simulink model "FOC_PMSM_JugandonoslaConDong_cris_v13"  (R2019b)
settings: Solver=VariableStepAuto  StartTime=0  StopTime=1.5  FixedStep=1/fs/4  MaxStep=1/fs/2  RelTol=1e-7  EnableMultiTasking=on
InitFcn:
  | Motor_parameters_Lsrpm7fw
undefined symbols (not defined in the file): c2, DiscIntNeverNeededParam, fs, Iphmax, J, Ki1, Ki2, Ki3, Ki_pll, Kp1, Kp2, Kp3, Kp_pll, Ld, Lndd_ini, Lndmpm, Lq, Npp, Omegae_ini, Rs, sigbuilder_block, Tl_const, Trat, Vm, Vph, wo
libraries: simulink x2
settings Model: Creator=klu  LastModifiedBy=Kristina
settings DataIOCC: LimitDataPoints=on  SaveFormat=Array  SignalLoggingSaveFormat=ModelDataLogs  ReturnWorkspaceOutputs=off
settings OptimizationCC: BooleanDataType=off  ExpressionDepthLimit=2147483647  InitFltsAndDblsToZero=on  LifeSpan=inf
settings DebuggingCC: AlgebraicLoopMsg=none  SaveWithParameterizedLinksMsg=none  UnderspecifiedInitializationDetection=Classic  MergeDetectMultiDrivingBlocksExec=none  SignalResolutionControl=TryResolveAllWithWarning  MultiTaskDSMMsg=warning  MultiTaskCondExecSysMsg=none  FcnCallInpInsideContextMsg=warning  StateNameClashWarn=warning  SFUnexpectedBacktrackingDiag=warning  SFNoUnconditionalDefaultTransitionDiag=warning  SFExecutionAtInitializationDiag=none  ArithmeticOperatorsInVariantConditions=warning
settings HardwareCC: ProdBitPerPointer=32  ProdBitPerSizeT=32  ProdBitPerPtrDiffT=32  ProdLargestAtomicFloat=None  ProdIntDivRoundTo=Undefined  ProdEndianess=Unspecified  ProdWordSize=32  ProdHWDeviceType=32-bit Generic
settings ModelReferenceCC: PropagateSignalLabelsOutOfModel=off
settings SFSimCC: SimUseLocalCustomCode=off  CustomCodeUndefinedFunction=UseInterfaceOnly
settings RTWCC: RTWUseLocalCustomCode=off
settings CodeAppCC: StateflowObjectComments=on
settings GRTTargetCC: TargetFcnLib=ansi_tfl_tmw.mat  TargetLangStandard=C89/C90 (ANSI)  GeneratePreprocessorConditionals=Disable all  CombineOutputUpdateFcns=off  GRTInterface=on
settings ConfigComp: CovMetricSettings=dw  CovHtmlReporting=on  CovSaveCumulativeToWorkspaceVar=on  CovSaveSingleToWorkspaceVar=on  CovExternalEMLEnable=off  CovSFcnEnable=off

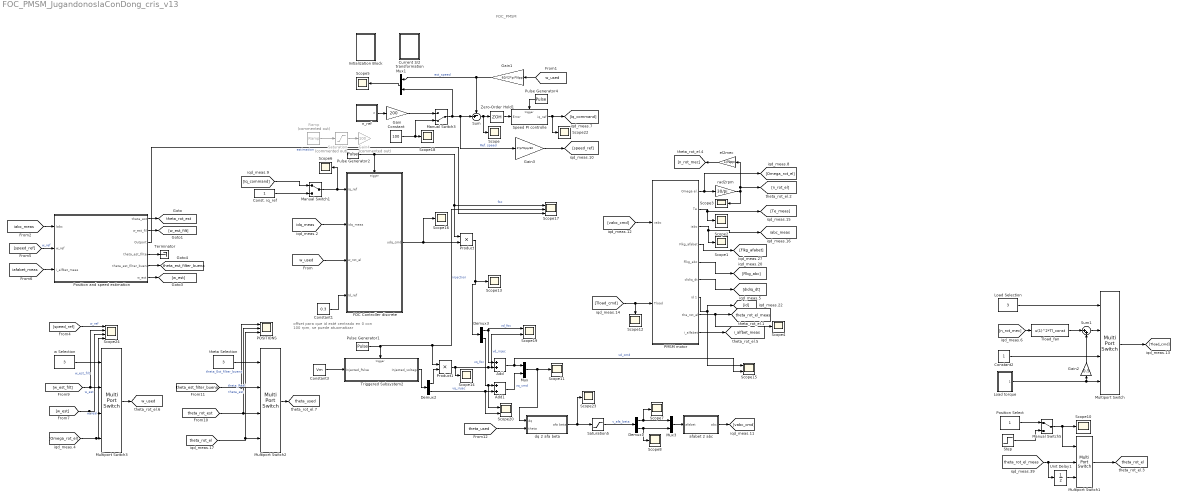
== system FOC_PMSM_JugandonoslaConDong_cris_v13 ==
  note: offset para que id esté centrado
      | en 0 con 100 rpm, se puede atuomatizar
  note: FOC_PMSM
  Add : Sum
  Add1 : Sum
  Const. iq_ref : Constant
  Constant : Constant  Value=100
  Constant1 : Constant  Value=0.3
  Constant2 : Constant
  Constant3 : Constant  Value=Vm
  Current 3/2 transformation : Subsystem
      mask Display:
      | plot([0.1000    0.1357    0.1714    0.2071    0.2429    0.2786    0.3143    0.3500    0.3857    0.4214 0.4571    0.4929    0.5286    0.5643    0.6000]-0.05,0.4+0.6*[0.5000    0.5868    0.6564    0.6950    0.6950    0.6564    0.5868    0.5000    0.4132    0.3436 0.3050    0.3050    0.3436    0.4132    0.5000])
      | 
      | plot([0.1,0.9],[0.1,0.9])
      | 
      | plot([0.5,0.9],0.3*[1 1])
  Demux1 : Demux  Outputs=2
  Demux2 : Demux  Outputs=2
  Demux3 : Demux  Outputs=2
  FOC Controller discrete : Subsystem
  Gain : Gain  Gain=200
  Gain1 : Gain  Gain=60/(2*pi*Npp)
  Gain2 : Gain  Gain=0.5
  Gain3 : Gain  Gain=2*pi*Npp/60
  Gain4 : Gain  Commented=on  Gain=100
  Initialization Block : Subsystem  mask{init_in=Motor_parameters_Lsrpm7fw}
      mask prompts: init_in "Enter Initialization Script:"
      mask init:
      | aaa =3;
      mask Callback init_in:
      | init_script=get_param(gcb,'MaskValueString');
      | %eval(init_script);
      | %set_param(gcs,'PreLoadFcn',init_script)
      | set_param(gcs,'InitFcn',init_script)
      | 
      | % Change the parameters here;
      | Ld               = Ld;
      | Lq               = Ld;
  Load Selection : Constant  Value=3
  Load torque : Subsystem
  Manual Switch1 : ManualSwitch
  Manual Switch3 : ManualSwitch  CurrentSetting=0
  Manual Switch5 : ManualSwitch
  Multiport Switch : MultiPortSwitch
  Multiport Switch1 : MultiPortSwitch  Inputs=2
  Multiport Switch2 : MultiPortSwitch
  Multiport Switch3 : MultiPortSwitch
  Mux : Mux  Inputs=2
  Mux1 : Mux  Inputs=2
  Mux3 : Mux  Inputs=2
  PMSM motor : Subsystem
  POSITIONS : Scope  NumInputPorts=3
  Position Select : Constant
  Position and speed estimation : Subsystem  TreatAsAtomicUnit=on
  Product : Product
  Product1 : Product
  Pulse Generator1 : DiscretePulseGenerator  PulseType=Time based  Period=2/fs  PulseWidth=50
  Pulse Generator2 : DiscretePulseGenerator  PulseType=Time based  Period=2/fs  PulseWidth=50  PhaseDelay=1/fs
  Pulse Generator4 : DiscretePulseGenerator  PulseType=Time based  Period=2/fs  PulseWidth=50  PhaseDelay=1/fs
  Ramp : simulink/Sources/Ramp  Commented=on  slope=0.5  start=0  InitialOutput=0.2
  Saturation : Saturate  Commented=on  UpperLimit=1
  Saturation5 : Saturate  UpperLimit=Vph  LowerLimit=-Vph
  Scope{,1..8,10..14,16,18,22..23} (18 alike) : Scope
  Scope15 : Scope  NumInputPorts=2
  Scope17 : Scope  NumInputPorts=3
  Scope19 : Scope  NumInputPorts=2
  Scope20 : Scope  NumInputPorts=2
  Scope24 : Scope  NumInputPorts=4
  Speed PI controlle : Subsystem
  Step : Step  Time=0  Before=1  After=2  SampleTime=0
  Sum : Sum  Inputs=-+|
  Sum1 : Sum  Inputs=|++
  Terminator : Terminator
  Tload_fan : Fcn  Expr=u(1)^2*Tl_const
  Triggered Subsystem2 : Subsystem  TreatAsAtomicUnit=on
  Unit Delay1 : UnitDelay  SampleTime=(1/fs)*4  HasFrameUpgradeWarning=on
  Zero-Order Hold1 : ZeroOrderHold  SampleTime=1/5e3
  afabet 2 abc : Subsystem
  dq 2 afa beta : Subsystem
  el2mec : Gain  Gain=1/Npp
  n_ref : Subsystem  Tag=STV Subsys  LoadFcn=sigbuilder_block('load');  StartFcn=sigbuilder_block('start');  StopFcn=sigbuilder_block('stop');  ClipboardFcn=sigbuilder_block('clipboard');  mask(Sigbuilder block){tuvar=[0:10]}
      mask help: Sigbuilder GUI
      mask init:
      | if ~strcmp(get_param(bdroot(gcbh),'SimulationStatus'),'stopped') tuvar = sigbuilder_block('maskInit'); end
      settings: CopyFcn=sigbuilder_block('copy');  DeleteFcn=sigbuilder_block('delete');  ModelCloseFcn=sigbuilder_block('modelClose');  PreSaveFcn=sigbuilder_block('preSave');  PauseFcn=sigbuilder_block('pause')  ContinueFcn=sigbuilder_block('continue')  NameChangeFcn=sigbuilder_block('namechange');  OpenFcn=sigbuilder_block('open',[72.75 116.25 550.5 363.75 ]);  CloseFcn=sigbuilder_block('close');
      mask Display: plot(0, 0, 100, 100,[2, 2, 32, 32, 2], [68, 8, 8, 68, 68],[32, 2], [38, 38], [32, 19, 2],[53, 60, 44], [32, 17, 17, 2],[16, 16, 31, 31]);txt = getActiveGroup(gcbh);text(2, 100, txt,'verticalAlignment', 'top');
  rad2rpm : Gain  Gain=30/pi
  theta Selection : Constant  Value=3
  w Selection : Constant  Value=3
  tag scope: i_alfbet_meas=global, iabc_meas=global, theta_est_filter_buena=global, theta_rot_el=global, theta_rot_el_meas=global, theta_rot_est=global, theta_used=global, w_used=global
  wires:
  Mux1/1 -> Scope5/1
  Sum/1 -> Scope/1, Zero-Order Hold1/1
  Manual Switch1/1 -> Scope6/1, FOC Controller discrete/1(iq_ref)
  Const. iq_ref/1 -> Manual Switch1/2
  Zero-Order Hold1/1 -> Speed PI controlle/1(Error)
  Constant/1 -> Manual Switch3/2, Scope18/1
  Manual Switch3/1 -> Mux1/2, Gain3/1, Sum/2  "Ref. speed"
  [idq_meas] -> FOC Controller discrete/2(idq_meas)
  Constant2/1 -> Multiport Switch/3
  Load torque/1(T_load) -> Multiport Switch/4, Gain2/1
  Multiport Switch/1 -> [Tload_cmd]
  [n_rot_mec] -> Tload_fan/1
  Load Selection/1 -> Multiport Switch/1
  [theta_rot_el_meas] -> Unit Delay1/1, Multiport Switch1/2
  Multiport Switch1/1 -> [theta_rot_el]
  Position Select/1 -> Manual Switch5/1
  Step/1 -> Manual Switch5/2
  Manual Switch5/1 -> Multiport Switch1/1, Scope10/1
  n_ref/1(n) -> Gain/1
  Gain/1 -> Manual Switch3/1
  Sum1/1 -> Multiport Switch/2
  Tload_fan/1 -> Sum1/1
  Pulse Generator4/1 -> Speed PI controlle/Trigger
  Constant1/1 -> FOC Controller discrete/4(Id_ref)
  Gain2/1 -> Sum1/2
  Unit Delay1/1 -> Multiport Switch1/3
  [vabc_cmd] -> PMSM motor/1(vabc)
  rad2rpm/1 -> el2mec/1, [n_rot_el], Scope3/1
  [Tload_cmd] -> PMSM motor/2(Tload), Scope12/1
  Demux1/2 -> Mux3/2, Scope8/1
  Demux1/1 -> Scope7/1, Mux3/1
  Saturation5/1 -> Demux1/1  "v_afa_beta"
  afabet 2 abc/1(abc) -> [vabc_cmd]
  Mux3/1 -> afabet 2 abc/1(afabet)
  el2mec/1 -> [n_rot_mec]
  Speed PI controlle/1(iq_ref) -> [Iq_command], Scope22/1
  [Iq_command] -> Manual Switch1/1
  Position and speed estimation/2(w_est_fil) -> [w_est_filt]
  Position and speed estimation/1(theta_est) -> [theta_rot_est]
  [iabc_meas] -> Position and speed estimation/1(Iabc)
  Gain1/1 -> Mux1/1, Sum/1  "est_speed"
  Gain3/1 -> [speed_ref]
  dq 2 afa beta/1(afa beta) -> Scope23/1, Saturation5/1
  [theta_used] -> dq 2 afa beta/2(theta)
  Constant3/1 -> Triggered Subsystem2/1(Injected_Pulse)
  FOC Controller discrete/1(udq_cmd) -> Product/2, Scope16/1
  Pulse Generator2/1 -> Product/1, Scope17/1, FOC Controller discrete/Trigger  "foc"
  Product/1 -> Scope13/1, Demux3/1
  Pulse Generator1/1 -> Scope17/2, Product1/1, Triggered Subsystem2/Trigger  "injection"
  Product1/1 -> Scope19/2, Add/2, Scope14/1  "vd_injec"
  Position and speed estimation/3(Outport) -> Scope17/3  "estimation"
  Triggered Subsystem2/1("Injected_voltage ") -> Demux2/1
  Demux2/1 -> Product1/2
  Demux3/1 -> Add/1, Scope19/1  "vd_foc"
  Demux2/2 -> Scope20/2, Add1/2  "vq_injec"
  Demux3/2 -> Scope20/1, Add1/1  "vq_foc"
  Add1/1 -> Mux/2  "vq_cmd"
  Mux/1 -> dq 2 afa beta/1(dq), Scope11/1
  Add/1 -> Scope15/2, Mux/1  "vd_cmd"
  Ramp/1 -> Saturation/1
  Saturation/1 -> Gain4/1
  PMSM motor/1(Omega el.) -> [Omega_rot_el], rad2rpm/1
  PMSM motor/2(Te) -> [Te_meas], Scope2/1
  PMSM motor/3(iabc) -> Scope1/1, [iabc_meas]
  PMSM motor/8(the_rot_el) -> Scope4/1, [theta_rot_el_meas]
  PMSM motor/7(id 1) -> [id], Scope15/1
  PMSM motor/6(didiq_dt) -> [didiq_dt]
  PMSM motor/5(Flkg_abc) -> [Flkg_abc]
  PMSM motor/4(Flkg_afabet) -> [Flkg_afabet]
  Position and speed estimation/4(theta_est_filter) -> Terminator/1
  Position and speed estimation/5(theta_est_filter_buena) -> [theta_est_filter_buena]
  PMSM motor/9(i_alfabet) -> [i_alfbet_meas]
  [iafabet_meas] -> Position and speed estimation/3(i_alfbet_meas)
  Position and speed estimation/6(w_est) -> [w_est]
  [w_used] -> Gain1/1
  [w_est_filt] -> Scope24/2, Multiport Switch3/2  "w_est_filt"
  [Omega_rot_el] -> Scope24/4, Multiport Switch3/4  "w_real"
  Multiport Switch3/1 -> [w_used]
  theta Selection/1 -> Multiport Switch2/1
  [theta_est_filter_buena] -> POSITIONS/1, Multiport Switch2/2  "theta_Est_filter_buena"
  [theta_rot_est] -> POSITIONS/2, Multiport Switch2/3  "theta_est"
  [theta_rot_el] -> POSITIONS/3, Multiport Switch2/4  "theta_Real"
  Multiport Switch2/1 -> [theta_used]
  w Selection/1 -> Multiport Switch3/1
  [w_est] -> Scope24/3, Multiport Switch3/3  "w_est"
  [speed_ref] -> Scope24/1  "w_ref"
  [speed_ref] -> Position and speed estimation/2(w_ref)  "w_ref"
  [w_used] -> FOC Controller discrete/3(w_rot_el)

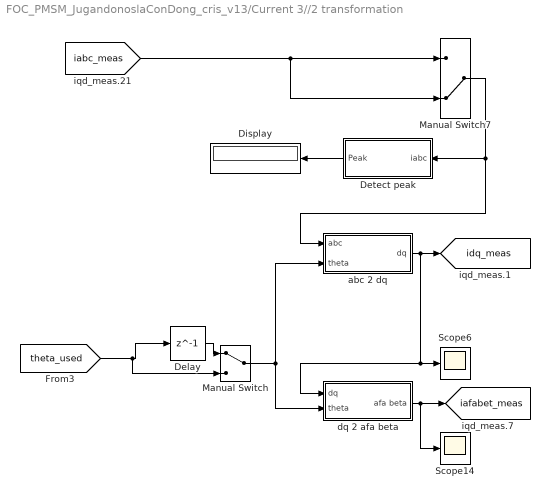
== system FOC_PMSM_JugandonoslaConDong_cris_v13/Current 3//2 transformation ==
  Delay : Delay  DelayLength=1
  Detect peak : Subsystem
  Display : Display
  Manual Switch : ManualSwitch
  Manual Switch7 : ManualSwitch  CurrentSetting=0
  Scope14 : Scope
  Scope6 : Scope
  abc 2 dq : Subsystem
  dq 2 afa beta : Subsystem
  tag scope: iafabet_meas=global, idq_meas=global
  wires:
  abc 2 dq/1(dq) -> [idq_meas], Scope6/1, dq 2 afa beta/1(dq)
  dq 2 afa beta/1(afa beta) -> [iafabet_meas], Scope14/1
  Manual Switch7/1 -> abc 2 dq/1(abc), Detect peak/1(iabc)
  Detect peak/1(Peak) -> Display/1
  [iabc_meas] -> Manual Switch7/1, Manual Switch7/2
  Manual Switch/1 -> abc 2 dq/2(theta), dq 2 afa beta/2(theta)
  Delay/1 -> Manual Switch/1
  [theta_used] -> Manual Switch/2, Delay/1

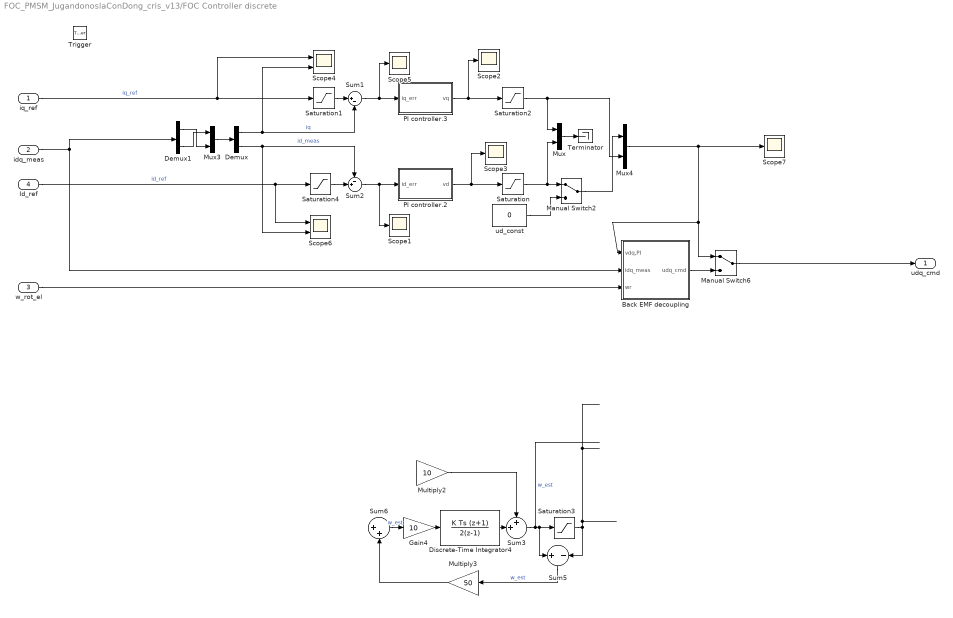
== system FOC_PMSM_JugandonoslaConDong_cris_v13/FOC Controller discrete ==
  iq_ref : Inport
  idq_meas : Inport  Port=2
  w_rot_el : Inport  Port=3
  Id_ref : Inport  Port=4
  Trigger : TriggerPort  VariantControl=(inherit)
  Back EMF decoupling : Subsystem
  Demux : Demux  Outputs=2
  Demux1 : Demux  Outputs=2
  Discrete-Time Integrator4 : DiscreteIntegrator  IntegratorMethod=Integration: Trapezoidal  gainval=1  SampleTime=-1  ICPrevOutput=DiscIntNeverNeededParam  ICPrevScaledInput=DiscIntNeverNeededParam
  Gain4 : Gain  Gain=10
  Manual Switch2 : ManualSwitch
  Manual Switch6 : ManualSwitch
  Multiply2 : Gain  Gain=10
  Multiply3 : Gain  Gain=50
  Mux : Mux  Inputs=2
  Mux3 : Mux  Inputs=2
  Mux4 : Mux  Inputs=2
  PI controller.2 : Subsystem
  PI controller.3 : Subsystem
  Saturation : Saturate  UpperLimit=Vph  LowerLimit=-Vph
  Saturation1 : Saturate  UpperLimit=Iphmax  LowerLimit=-Iphmax
  Saturation2 : Saturate  UpperLimit=Vph  LowerLimit=-Vph
  Saturation3 : Saturate  UpperLimit=110*Npp*2*pi/60
  Saturation4 : Saturate  UpperLimit=Iphmax  LowerLimit=-Iphmax
  Scope{1..3,5,7} (5 alike) : Scope
  Scope4 : Scope  NumInputPorts=2
  Scope6 : Scope  NumInputPorts=2
  Sum1 : Sum  Inputs=|+-
  Sum2 : Sum  Inputs=-+|
  Sum3 : Sum  Inputs=++|
  Sum5 : Sum  Inputs=+|-
  Sum6 : Sum  Inputs=|++
  Terminator : Terminator
  ud_const : Constant  Value=0
  udq_cmd : Outport  VectorParamsAs1DForOutWhenUnconnected=off
  wires:
  Saturation4/1 -> Sum2/2
  Saturation/1 -> Mux/2, Manual Switch2/1
  Mux/1 -> Terminator/1
  PI controller.3/1(vq) -> Scope2/1, Saturation2/1
  Demux/1 -> Scope4/2, Sum1/2  "iq"
  PI controller.2/1(vd) -> Saturation/1, Scope3/1
  Demux/2 -> Scope6/2, Sum2/1  "id_meas"
  Sum1/1 -> Scope5/1, PI controller.3/1(iq_err)
  iq_ref/1 -> Scope4/1, Saturation1/1  "iq_ref"
  Sum2/1 -> Scope1/1, PI controller.2/1(id_err)
  Id_ref/1 -> Scope6/1, Saturation4/1  "id_ref"
  Saturation1/1 -> Sum1/1
  Saturation2/1 -> Mux/1, Mux4/2
  Manual Switch2/1 -> Mux4/1
  ud_const/1 -> Manual Switch2/2
  Demux1/2 -> Mux3/1
  Demux1/1 -> Mux3/2
  w_rot_el/1 -> Back EMF decoupling/3(wr)
  Back EMF decoupling/1(udq_cmd) -> Manual Switch6/2
  Mux4/1 -> Scope7/1, Manual Switch6/1, Back EMF decoupling/1(vdq,PI)
  Mux3/1 -> Demux/1
  idq_meas/1 -> Demux1/1, Back EMF decoupling/2(idq_meas)
  Manual Switch6/1 -> udq_cmd/1
  Sum3/1 -> Sum5/1, Saturation3/1  "w_est"
  Saturation3/1 -> Sum5/2
  Sum6/1 -> Gain4/1  "w_est"
  Multiply3/1 -> Sum6/2
  ? -> Multiply2/1, Sum6/1  "theta_er"
  Gain4/1 -> Discrete-Time Integrator4/1
  Multiply2/1 -> Sum3/1
  Discrete-Time Integrator4/1 -> Sum3/2
  Sum5/1 -> Multiply3/1  "w_est"

== system FOC_PMSM_JugandonoslaConDong_cris_v13/Initialization Block ==

== system FOC_PMSM_JugandonoslaConDong_cris_v13/Load torque ==
  Add : Sum  Inputs=+++
  Scope2 : Scope
  Step Load torque 1 : Step  Time=0.7  After=Trat  SampleTime=0
  Step Load torque2 : Step  Time=2.5  After=-Trat  SampleTime=0
  Tload : Constant  Value=0
  T_load : Outport  VectorParamsAs1DForOutWhenUnconnected=off
  wires:
  Tload/1 -> Add/1
  Step Load torque 1/1 -> Add/2
  Step Load torque2/1 -> Add/3
  Add/1 -> T_load/1, Scope2/1

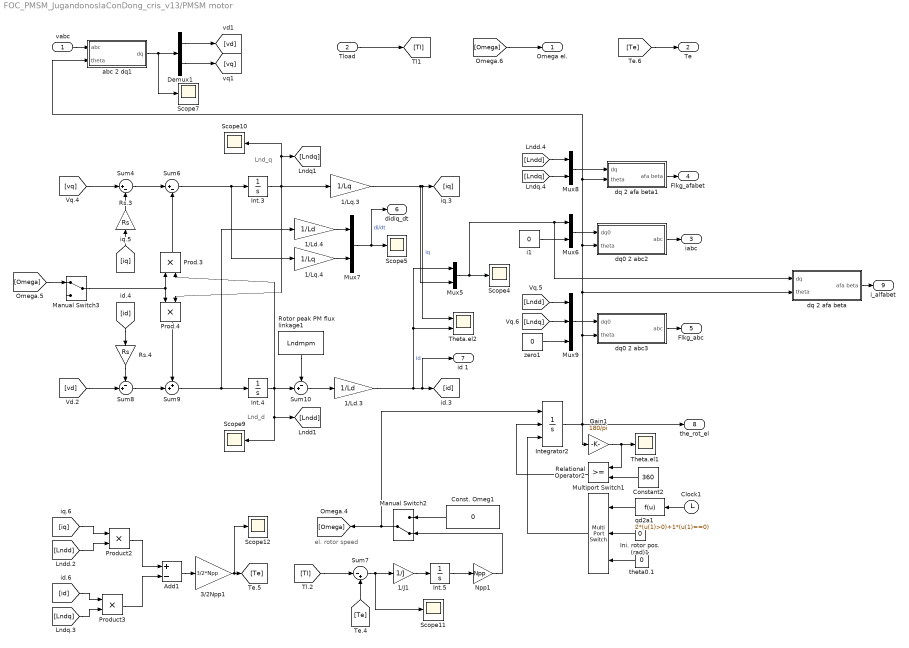
== system FOC_PMSM_JugandonoslaConDong_cris_v13/PMSM motor ==
  note: Lnd_d
  note: el. rotor speed
  note: Lnd_q
  vabc : Inport
  Tload : Inport  Port=2
  1/J1 : Gain  Gain=1/J
  1/Ld.3 : Gain  Gain=1/Ld
  1/Ld.4 : Gain  Gain=1/Ld
  1/Lq.3 : Gain  Gain=1/Lq
  1/Lq.4 : Gain  Gain=1/Lq
  3/2Npp1 : Gain  Gain=3/2*Npp
  Add1 : Sum  Inputs=+-
  Clock1 : Clock
  Const. Omeg1 : Constant  Value=0
  Constant2 : Constant  Value=360
  Demux1 : Demux  Outputs=2
  Gain1 : Gain  Gain=180/pi
  Ini. rotor pos. (rad)1 : Constant  Value=0
  Int.3 : Integrator
  Int.4 : Integrator  InitialCondition=Lndd_ini
  Int.5 : Integrator  InitialCondition=Omegae_ini/Npp
  Integrator2 : Integrator  ExternalReset=rising  InitialConditionSource=external  InitialCondition=pi/3
  Manual Switch2 : ManualSwitch  CurrentSetting=0
  Manual Switch3 : ManualSwitch
  Multiport Switch1 : MultiPortSwitch  Inputs=2
  Mux{5..8} (4 alike) : Mux  Inputs=2
  Mux9 : Mux  Inputs=3
  Npp1 : Gain  Gain=Npp
  Prod.3 : Product  RndMeth=Zero
  Prod.4 : Product  RndMeth=Zero
  Product2 : Product  RndMeth=Zero
  Product3 : Product  RndMeth=Zero
  Relational Operator2 : RelationalOperator  OutDataTypeStr=boolean  RndMeth=Nearest
  Rotor peak PM flux linkage1 : Constant  Value=Lndmpm
  Rs.3 : Gain  Gain=Rs
  Rs.4 : Gain  Gain=Rs
  Scope{4..5,7,9..12} (7 alike) : Scope
  Sum10 : Sum  Inputs=-+|
  Sum4 : Sum  Inputs=|+-
  Sum6 : Sum  Inputs=|+-
  Sum7 : Sum  Inputs=|-+
  Sum8 : Sum  Inputs=-+|
  Sum9 : Sum  Inputs=++|
  Theta.el1 : Scope
  Theta.el2 : Scope  NumInputPorts=2
  abc 2 dq1 : Subsystem
  dq 2 afa beta : Subsystem
  dq 2 afa beta1 : Subsystem
  dq0 2 abc2 : Subsystem
  dq0 2 abc3 : Subsystem
  i1 : Constant  Value=0
  qd2a1 : Fcn  Expr=2*(u(1)>0)+1*(u(1)==0)
  theta0.1 : Constant  Value=0
  zero1 : Constant  Value=0
  Omega el. : Outport  VectorParamsAs1DForOutWhenUnconnected=off
  Te : Outport  Port=2  VectorParamsAs1DForOutWhenUnconnected=off
  iabc : Outport  Port=3  VectorParamsAs1DForOutWhenUnconnected=off
  Flkg_afabet : Outport  Port=4  VectorParamsAs1DForOutWhenUnconnected=off
  Flkg_abc : Outport  Port=5  VectorParamsAs1DForOutWhenUnconnected=off
  didiq_dt : Outport  Port=6  VectorParamsAs1DForOutWhenUnconnected=off
  id 1 : Outport  Port=7  VectorParamsAs1DForOutWhenUnconnected=off
  the_rot_el : Outport  Port=8  VectorParamsAs1DForOutWhenUnconnected=off
  i_alfabet : Outport  Port=9  VectorParamsAs1DForOutWhenUnconnected=off
  wires:
  Sum4/1 -> Sum6/1
  [vd] -> Sum8/2
  Mux5/1 -> Scope4/1, dq 2 afa beta/1(dq), Mux6/1
  Mux7/1 -> didiq_dt/1, Scope5/1  "di/dt"
  Int.3/1 -> 1/Lq.3/1, Prod.4/2, Scope10/1, [Lndq]
  abc 2 dq1/1(dq) -> Demux1/1, Scope7/1
  Tload/1 -> [Tl]
  Rs.3/1 -> Sum4/2
  1/Ld.4/1 -> Mux7/1
  Integrator2/1 -> the_rot_el/1, dq 2 afa beta/2(theta), dq0 2 abc2/2(theta), dq 2 afa beta1/2(theta), abc 2 dq1/2(theta), dq0 2 abc3/2(theta), Gain1/1
  Prod.4/1 -> Sum9/1
  [Lndq] -> Product3/2
  1/J1/1 -> Int.5/1
  [Lndd] -> Mux8/1
  [Te] -> Te/1
  [iq] -> Rs.3/1
  Sum10/1 -> 1/Ld.3/1
  Rotor peak PM flux linkage1/1 -> Sum10/1
  Int.4/1 -> [Lndd], Scope9/1, Sum10/2, Prod.3/2
  Int.5/1 -> Npp1/1
  Sum8/1 -> Sum9/2
  Add1/1 -> 3/2Npp1/1
  3/2Npp1/1 -> Scope12/1, [Te]
  Product3/1 -> Add1/2
  Demux1/2 -> [vq]
  Prod.3/1 -> Sum6/2
  1/Lq.3/1 -> Theta.el2/1, [iq], Mux5/2  "iq"
  1/Ld.3/1 -> Theta.el2/2, Mux5/1, id 1/1, [id]  "id"
  [Omega] -> Omega el./1
  [Omega] -> Manual Switch3/1
  1/Lq.4/1 -> Mux7/2
  [vq] -> Sum4/1
  Npp1/1 -> Manual Switch2/2
  Gain1/1 -> Theta.el1/1, Relational Operator2/1
  dq0 2 abc2/1(abc) -> iabc/1
  [Te] -> Sum7/2
  Ini. rotor pos. (rad)1/1 -> Multiport Switch1/2
  Sum6/1 -> Int.3/1, 1/Lq.4/1
  Manual Switch3/1 -> Prod.4/1, Prod.3/1
  i1/1 -> Mux6/2
  dq0 2 abc3/1(abc) -> Flkg_abc/1
  Relational Operator2/1 -> Integrator2/2
  [Lndq] -> Mux9/2
  Multiport Switch1/1 -> Integrator2/3
  Constant2/1 -> Relational Operator2/2
  [Lndd] -> Product2/2
  [iq] -> Product2/1
  [id] -> Product3/1
  Product2/1 -> Add1/1
  Clock1/1 -> qd2a1/1
  [id] -> Rs.4/1
  vabc/1 -> abc 2 dq1/1(abc)
  Mux6/1 -> dq0 2 abc2/1(dq0)
  Demux1/1 -> [vd]
  Const. Omeg1/1 -> Manual Switch2/1
  Rs.4/1 -> Sum8/1
  [Lndd] -> Mux9/1
  theta0.1/1 -> Multiport Switch1/3
  Sum7/1 -> Scope11/1, 1/J1/1
  [Lndq] -> Mux8/2
  Mux9/1 -> dq0 2 abc3/1(dq0)
  Manual Switch2/1 -> Integrator2/1, [Omega]
  Mux8/1 -> dq 2 afa beta1/1(dq)
  dq 2 afa beta1/1(afa beta) -> Flkg_afabet/1
  qd2a1/1 -> Multiport Switch1/1
  zero1/1 -> Mux9/3
  [Tl] -> Sum7/1
  Sum9/1 -> Int.4/1, 1/Ld.4/1
  dq 2 afa beta/1(afa beta) -> i_alfabet/1

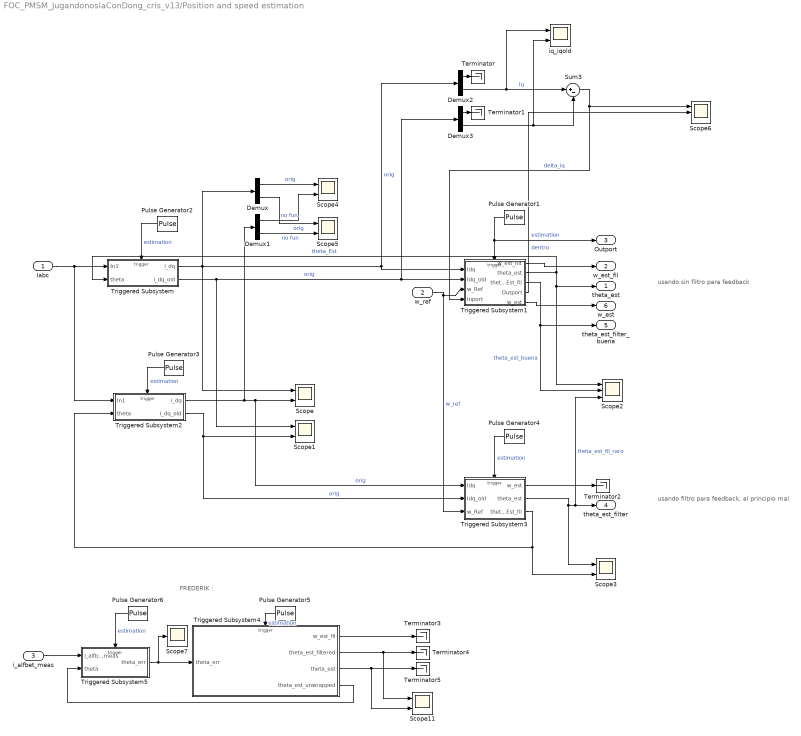
== system FOC_PMSM_JugandonoslaConDong_cris_v13/Position and speed estimation ==
  note: FREDERIK :
  note: usando filtro para feedback, al principio mal
  note: usando sin filtro para feedback
  Iabc : Inport
  w_ref : Inport  Port=2
  i_alfbet_meas : Inport  Port=3
  Demux{,1..3} (4 alike) : Demux  Outputs=2
  Pulse Generator1 : DiscretePulseGenerator  PulseType=Time based  Period=2/fs  PulseWidth=50
  Pulse Generator2 : DiscretePulseGenerator  PulseType=Time based  Period=1/fs  PulseWidth=50
  Pulse Generator3 : DiscretePulseGenerator  PulseType=Time based  Period=1/fs  PulseWidth=50
  Pulse Generator4 : DiscretePulseGenerator  PulseType=Time based  Period=2/fs  PulseWidth=50  PhaseDelay=1/fs
  Pulse Generator5 : DiscretePulseGenerator  PulseType=Time based  Period=2/fs  PulseWidth=50  PhaseDelay=1/fs
  Pulse Generator6 : DiscretePulseGenerator  PulseType=Time based  Period=1/fs  PulseWidth=50
  Scope{,1,3..5,11} (6 alike) : Scope  NumInputPorts=2
  Scope2 : Scope  NumInputPorts=3
  Scope6 : Scope  NumInputPorts=3
  Scope7 : Scope
  Sum3 : Sum  Inputs=|+-
  Terminator{,1..5} (6 alike) : Terminator
  Triggered Subsystem : Subsystem  TreatAsAtomicUnit=on
  Triggered Subsystem1 : Subsystem  TreatAsAtomicUnit=on
  Triggered Subsystem2 : Subsystem  TreatAsAtomicUnit=on
  Triggered Subsystem3 : Subsystem  TreatAsAtomicUnit=on
  Triggered Subsystem4 : Subsystem  TreatAsAtomicUnit=on
  Triggered Subsystem5 : Subsystem  TreatAsAtomicUnit=on
  iq_iqold : Scope  NumInputPorts=2
  theta_est : Outport
  w_est_fil : Outport  Port=2
  Outport : Outport  Port=3
  theta_est_filter : Outport  Port=4
  theta_est_filter_buena : Outport  Port=5
  w_est : Outport  Port=6
  wires:
  Pulse Generator1/1 -> Triggered Subsystem1/Trigger, Outport/1  "estimation"
  Triggered Subsystem1/1(w_est_filt) -> w_est_fil/1
  Triggered Subsystem/2(i_dq_old) -> Scope1/1, Demux3/1, Triggered Subsystem1/2(Idq_old)  "orig"
  Triggered Subsystem1/2(theta_est) -> Scope2/1, theta_est/1, Triggered Subsystem/2(theta)  "theta_Est"
  Triggered Subsystem/1(i_dq) -> Scope/1, Demux/1, Demux2/1, Triggered Subsystem1/1(Idq)  "orig"
  w_ref/1 -> Triggered Subsystem3/3(w_Ref), Triggered Subsystem1/3(w_Ref)  "w_ref"
  Pulse Generator2/1 -> Triggered Subsystem/Trigger  "estimation"
  Triggered Subsystem1/3(theta_Est_fil) -> theta_est_filter_buena/1, Scope2/2  "theta_est_buena"
  Pulse Generator3/1 -> Triggered Subsystem2/Trigger  "estimation"
  Demux/1 -> Scope4/1  "orig"
  Demux1/1 -> Scope4/2  "no fun"
  Demux/2 -> Scope5/1  "orig"
  Demux1/2 -> Scope5/2  "no fun"
  Pulse Generator4/1 -> Triggered Subsystem3/Trigger  "estimation"
  Triggered Subsystem3/3(theta_Est_fil) -> Triggered Subsystem2/2(theta), Scope3/2
  Triggered Subsystem2/2(i_dq_old) -> Triggered Subsystem3/2(Idq_old), Scope1/2  "orig"
  Triggered Subsystem2/1(i_dq) -> Triggered Subsystem3/1(Idq), Scope/2, Demux1/1  "orig"
  Triggered Subsystem3/2(theta_est) -> Scope3/1, Scope2/3, theta_est_filter/1  "theta_est_fil_raro"
  Triggered Subsystem3/1(w_est) -> Terminator2/1
  Demux2/1 -> Terminator/1
  Demux3/1 -> Terminator1/1
  Demux2/2 -> iq_iqold/1, Sum3/1  "Iq"
  Demux3/2 -> iq_iqold/2, Sum3/2
  Sum3/1 -> Triggered Subsystem1/4(Inport), Scope6/1  "delta_iq"
  Triggered Subsystem1/4(Outport) -> Scope6/2  "dentro"
  Iabc/1 -> Triggered Subsystem2/1(In1), Triggered Subsystem/1(In1)
  Triggered Subsystem4/3(theta_est) -> Terminator5/1, Scope11/2
  i_alfbet_meas/1 -> Triggered Subsystem5/1(i_alfbet_meas)
  Triggered Subsystem4/1(w_est_fil) -> Terminator3/1
  Triggered Subsystem4/2(theta_est_filtered) -> Terminator4/1, Scope11/1
  Pulse Generator5/1 -> Triggered Subsystem4/Trigger  "estimation"
  Pulse Generator6/1 -> Triggered Subsystem5/Trigger  "estimation"
  Triggered Subsystem5/1(theta_err) -> Scope7/1, Triggered Subsystem4/1(theta_err)
  Triggered Subsystem4/4(theta_est_unwrapped) -> Triggered Subsystem5/2(theta)
  Triggered Subsystem1/5(w_est) -> w_est/1

== system FOC_PMSM_JugandonoslaConDong_cris_v13/Speed PI controlle ==
  Error : Inport
  Trigger : TriggerPort  VariantControl=(inherit)
  Discrete-Time Integrator : DiscreteIntegrator  IntegratorMethod=Integration: Trapezoidal  SampleTime=-1  ICPrevOutput=DiscIntNeverNeededParam  ICPrevScaledInput=DiscIntNeverNeededParam
  Kp : Gain  Gain=Kp1
  Sum1 : Sum  Inputs=|++
  ki : Gain  Gain=Ki1
  iq_ref : Outport  VectorParamsAs1DForOutWhenUnconnected=off
  wires:
  Kp/1 -> Sum1/1
  ki/1 -> Discrete-Time Integrator/1
  Discrete-Time Integrator/1 -> Sum1/2
  Sum1/1 -> iq_ref/1
  Error/1 -> Kp/1, ki/1

== system FOC_PMSM_JugandonoslaConDong_cris_v13/Triggered Subsystem2 ==
  Injected_Pulse : Inport
  Trigger : TriggerPort  VariantControl=Variant
  Constant : Constant  Value=0
  Mux5 : Mux  Inputs=2
  Saturation3 : Saturate  UpperLimit=Vph  LowerLimit=-Vph
  "Injected_voltage " : Outport
  wires:
  Injected_Pulse/1 -> Mux5/1
  Constant/1 -> Mux5/2
  Mux5/1 -> Saturation3/1  "vdq_cmd_inj"
  Saturation3/1 -> "Injected_voltage "/1

== system FOC_PMSM_JugandonoslaConDong_cris_v13/afabet 2 abc ==
  afabet : Inport
  Constant : Constant  Value=0
  Mux1 : Mux  Inputs=2
  Mux2 : Mux  Inputs=3
  qd2a : Fcn  Expr=u(1)+u(3)
  qd2b : Fcn  Expr=u(1)*cos(2/3*pi)+u(2)*sin(2/3*pi)+u(3)
  qd2c : Fcn  Expr=u(1)*cos(2/3*pi)-u(2)*sin(2/3*pi)+u(3)
  abc : Outport  VectorParamsAs1DForOutWhenUnconnected=off
  wires:
  Constant/1 -> Mux1/2
  qd2c/1 -> Mux2/3
  afabet/1 -> Mux1/1
  Mux1/1 -> qd2c/1, qd2b/1, qd2a/1
  qd2a/1 -> Mux2/1
  qd2b/1 -> Mux2/2
  Mux2/1 -> abc/1

== system FOC_PMSM_JugandonoslaConDong_cris_v13/dq 2 afa beta ==
  dq : Inport
  theta : Inport  Port=2
  Mux1 : Mux  Inputs=2
  Mux2 : Mux  Inputs=2
  dq2afa : Fcn  Expr=u(1)*cos(u(3))-u(2)*sin(u(3))
  dq2beta : Fcn  Expr=u(1)*sin(u(3))+u(2)*cos(u(3))
  afa beta : Outport  VectorParamsAs1DForOutWhenUnconnected=off
  wires:
  Mux2/1 -> afa beta/1
  dq2beta/1 -> Mux2/2
  dq2afa/1 -> Mux2/1
  Mux1/1 -> dq2afa/1, dq2beta/1
  theta/1 -> Mux1/2
  dq/1 -> Mux1/1

== system FOC_PMSM_JugandonoslaConDong_cris_v13/n_ref ==
  Demux : Demux  Tag=STV Demux  Outputs=1
  FromWs : FromWorkspace  Tag=STV FromWs  VariableName=tuvar  SampleTime=0
      SigBuilderData=|
      | common.afterFinalStr = 'Extrapolate'
      | common.sampleTime = 0
      | dataSet.timeRange = [0 10]
      | dataSet.name = 'Group 1'
      | sbobj.Groups.Name = 'Group 1'
      | sbobj.Groups.Signals.Name = 'n'
      | sbobj.Groups.Signals.XData = [0 4 4 5 5 7 10]
      | sbobj.Groups.Signals.YData = [0.21 0.795 0.995 0.995 0.4 0.405 0.2]
  n : Outport  Tag=STV Outport  VectorParamsAs1DForOutWhenUnconnected=off
  wires:
  Demux/1 -> n/1
  FromWs/1 -> Demux/1

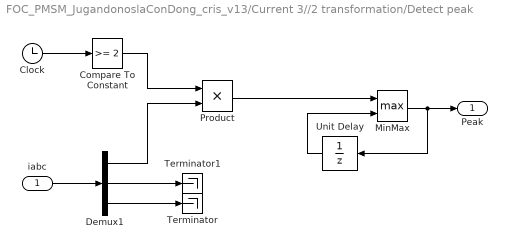
== system FOC_PMSM_JugandonoslaConDong_cris_v13/Current 3//2 transformation/Detect peak ==
  iabc : Inport
  Clock : Clock
  Compare To Constant : simulink/Logic and Bit Operations/Compare To Constant  relop=>=  const=2  OutDataTypeStr=uint8  ZeroCross=off
  Demux1 : Demux  Outputs=3
  MinMax : MinMax  Function=max  Inputs=2
  Product : Product  RndMeth=Zero
  Terminator : Terminator
  Terminator1 : Terminator
  Unit Delay : UnitDelay  SampleTime=1/5e3  HasFrameUpgradeWarning=on
  Peak : Outport  VectorParamsAs1DForOutWhenUnconnected=off
  wires:
  iabc/1 -> Demux1/1
  Demux1/3 -> Terminator/1
  Demux1/2 -> Terminator1/1
  Clock/1 -> Compare To Constant/1
  Compare To Constant/1 -> Product/1
  Demux1/1 -> Product/2
  MinMax/1 -> Peak/1, Unit Delay/1
  Product/1 -> MinMax/1
  Unit Delay/1 -> MinMax/2

== system FOC_PMSM_JugandonoslaConDong_cris_v13/Current 3//2 transformation/abc 2 dq ==
  abc : Inport
  theta : Inport  Port=2
  Mux1 : Mux  Inputs=2
  Mux2 : Mux  Inputs=2
  abc2d : Fcn  Expr=2/3*(u(1)*cos(u(4))+u(2)*cos(u(4)-2*pi/3)+u(3)*cos(u(4)-4*pi/3))
  abc2q : Fcn  Expr=-1*2/3*(u(1)*sin(u(4))+u(2)*sin(u(4)-2*pi/3)+u(3)*sin(u(4)-4*pi/3))
  dq : Outport  VectorParamsAs1DForOutWhenUnconnected=off
  wires:
  Mux2/1 -> dq/1
  abc2q/1 -> Mux2/2
  abc2d/1 -> Mux2/1
  Mux1/1 -> abc2q/1, abc2d/1
  theta/1 -> Mux1/2
  abc/1 -> Mux1/1

== system FOC_PMSM_JugandonoslaConDong_cris_v13/Current 3//2 transformation/dq 2 afa beta ==
  dq : Inport
  theta : Inport  Port=2
  Mux1 : Mux  Inputs=2
  Mux2 : Mux  Inputs=2
  dq2afa : Fcn  Expr=u(1)*cos(u(3))-u(2)*sin(u(3))
  dq2beta : Fcn  Expr=u(1)*sin(u(3))+u(2)*cos(u(3))
  afa beta : Outport  VectorParamsAs1DForOutWhenUnconnected=off
  wires:
  dq/1 -> Mux1/1
  theta/1 -> Mux1/2
  Mux1/1 -> dq2beta/1, dq2afa/1
  dq2afa/1 -> Mux2/1
  dq2beta/1 -> Mux2/2
  Mux2/1 -> afa beta/1

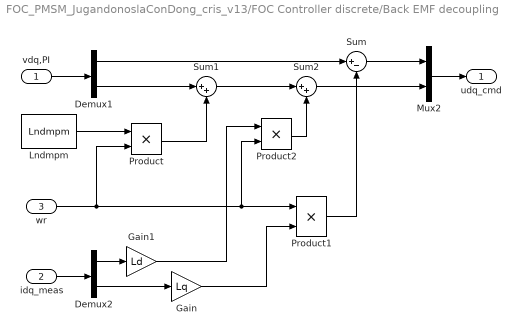
== system FOC_PMSM_JugandonoslaConDong_cris_v13/FOC Controller discrete/Back EMF decoupling ==
  vdq,PI : Inport
  idq_meas : Inport  Port=2
  wr : Inport  Port=3
  Demux1 : Demux  Outputs=2
  Demux2 : Demux  Outputs=2
  Gain : Gain  Gain=Lq
  Gain1 : Gain  Gain=Ld
  Lndmpm : Constant  Value=Lndmpm
  Mux2 : Mux  Inputs=2
  Product : Product  RndMeth=Zero
  Product1 : Product  RndMeth=Zero
  Product2 : Product  RndMeth=Zero
  Sum : Sum  Inputs=|+-
  Sum1 : Sum  Inputs=|++
  Sum2 : Sum  Inputs=|++
  udq_cmd : Outport  VectorParamsAs1DForOutWhenUnconnected=off
  wires:
  Mux2/1 -> udq_cmd/1
  vdq,PI/1 -> Demux1/1
  Demux1/1 -> Sum/1
  Sum/1 -> Mux2/1
  Demux1/2 -> Sum1/1
  idq_meas/1 -> Demux2/1
  wr/1 -> Product/2, Product1/1, Product2/2
  Product1/1 -> Sum/2
  Gain/1 -> Product1/2
  Demux2/2 -> Gain/1
  Lndmpm/1 -> Product/1
  Product/1 -> Sum1/2
  Sum1/1 -> Sum2/1
  Demux2/1 -> Gain1/1
  Gain1/1 -> Product2/1
  Product2/1 -> Sum2/2
  Sum2/1 -> Mux2/2

== system FOC_PMSM_JugandonoslaConDong_cris_v13/FOC Controller discrete/PI controller.2 ==
  id_err : Inport
  Discrete-Time Integrator : DiscreteIntegrator  IntegratorMethod=Integration: Trapezoidal  SampleTime=-1  ICPrevOutput=DiscIntNeverNeededParam  ICPrevScaledInput=DiscIntNeverNeededParam
  Kp : Gain  Gain=Kp2
  Sum1 : Sum  Inputs=|++
  ki : Gain  Gain=Ki2
  vd : Outport  VectorParamsAs1DForOutWhenUnconnected=off
  wires:
  Sum1/1 -> vd/1
  Discrete-Time Integrator/1 -> Sum1/2
  ki/1 -> Discrete-Time Integrator/1
  Kp/1 -> Sum1/1
  id_err/1 -> ki/1, Kp/1

== system FOC_PMSM_JugandonoslaConDong_cris_v13/FOC Controller discrete/PI controller.3 ==
  iq_err : Inport
  Discrete-Time Integrator : DiscreteIntegrator  IntegratorMethod=Integration: Trapezoidal  SampleTime=-1  ICPrevOutput=DiscIntNeverNeededParam  ICPrevScaledInput=DiscIntNeverNeededParam
  Kp : Gain  Gain=Kp3
  Sum1 : Sum  Inputs=|++
  ki : Gain  Gain=Ki3
  vq : Outport  VectorParamsAs1DForOutWhenUnconnected=off
  wires:
  Sum1/1 -> vq/1
  Discrete-Time Integrator/1 -> Sum1/2
  ki/1 -> Discrete-Time Integrator/1
  Kp/1 -> Sum1/1
  iq_err/1 -> ki/1, Kp/1

== system FOC_PMSM_JugandonoslaConDong_cris_v13/PMSM motor/abc 2 dq1 ==
  abc : Inport
  theta : Inport  Port=2
  Mux1 : Mux  Inputs=2
  Mux2 : Mux  Inputs=2
  abc2d : Fcn  Expr=-1*2/3*(u(1)*sin(u(4))+u(2)*sin(u(4)-2*pi/3)+u(3)*sin(u(4)-4*pi/3))
  abc2q : Fcn  Expr=2/3*(u(1)*cos(u(4))+u(2)*cos(u(4)-2*pi/3)+u(3)*cos(u(4)-4*pi/3))
  dq : Outport  VectorParamsAs1DForOutWhenUnconnected=off
  wires:
  Mux2/1 -> dq/1
  abc2d/1 -> Mux2/2
  abc2q/1 -> Mux2/1
  Mux1/1 -> abc2d/1, abc2q/1
  theta/1 -> Mux1/2
  abc/1 -> Mux1/1

== system FOC_PMSM_JugandonoslaConDong_cris_v13/PMSM motor/dq 2 afa beta ==
  dq : Inport
  theta : Inport  Port=2
  Mux1 : Mux  Inputs=2
  Mux2 : Mux  Inputs=2
  dq2afa : Fcn  Expr=u(1)*cos(u(3))-u(2)*sin(u(3))
  dq2beta : Fcn  Expr=u(1)*sin(u(3))+u(2)*cos(u(3))
  afa beta : Outport  VectorParamsAs1DForOutWhenUnconnected=off
  wires:
  Mux2/1 -> afa beta/1
  dq2beta/1 -> Mux2/2
  dq2afa/1 -> Mux2/1
  Mux1/1 -> dq2afa/1, dq2beta/1
  theta/1 -> Mux1/2
  dq/1 -> Mux1/1

== system FOC_PMSM_JugandonoslaConDong_cris_v13/PMSM motor/dq 2 afa beta1 ==
  dq : Inport
  theta : Inport  Port=2
  Mux1 : Mux  Inputs=2
  Mux2 : Mux  Inputs=2
  dq2afa : Fcn  Expr=u(1)*cos(u(3))-u(2)*sin(u(3))
  dq2beta : Fcn  Expr=u(1)*sin(u(3))+u(2)*cos(u(3))
  afa beta : Outport  VectorParamsAs1DForOutWhenUnconnected=off
  wires:
  dq/1 -> Mux1/1
  theta/1 -> Mux1/2
  Mux1/1 -> dq2beta/1, dq2afa/1
  dq2afa/1 -> Mux2/1
  dq2beta/1 -> Mux2/2
  Mux2/1 -> afa beta/1

== system FOC_PMSM_JugandonoslaConDong_cris_v13/PMSM motor/dq0 2 abc2 ==
  dq0 : Inport
  theta : Inport  Port=2
  Mux1 : Mux  Inputs=2
  Mux2 : Mux  Inputs=3
  qd2a : Fcn  Expr=u(1)*cos(u(4))-u(2)*sin(u(4))+u(3)
  qd2b : Fcn  Expr=u(1)*cos(u(4)-2/3*pi)-u(2)*sin(u(4)-2/3*pi)+u(3)
  qd2c : Fcn  Expr=u(1)*cos(u(4)+2/3*pi)-u(2)*sin(u(4)+2/3*pi)+u(3)
  abc : Outport  VectorParamsAs1DForOutWhenUnconnected=off
  wires:
  Mux2/1 -> abc/1
  qd2b/1 -> Mux2/2
  qd2a/1 -> Mux2/1
  Mux1/1 -> qd2b/1, qd2c/1, qd2a/1
  theta/1 -> Mux1/2
  dq0/1 -> Mux1/1
  qd2c/1 -> Mux2/3

== system FOC_PMSM_JugandonoslaConDong_cris_v13/PMSM motor/dq0 2 abc3 ==
  dq0 : Inport
  theta : Inport  Port=2
  Mux1 : Mux  Inputs=2
  Mux2 : Mux  Inputs=3
  qd2a : Fcn  Expr=u(1)*cos(u(4))-u(2)*sin(u(4))+u(3)
  qd2b : Fcn  Expr=u(1)*cos(u(4)-2/3*pi)-u(2)*sin(u(4)-2/3*pi)+u(3)
  qd2c : Fcn  Expr=u(1)*cos(u(4)+2/3*pi)-u(2)*sin(u(4)+2/3*pi)+u(3)
  abc : Outport  VectorParamsAs1DForOutWhenUnconnected=off
  wires:
  qd2c/1 -> Mux2/3
  dq0/1 -> Mux1/1
  theta/1 -> Mux1/2
  Mux1/1 -> qd2a/1, qd2c/1, qd2b/1
  qd2a/1 -> Mux2/1
  qd2b/1 -> Mux2/2
  Mux2/1 -> abc/1

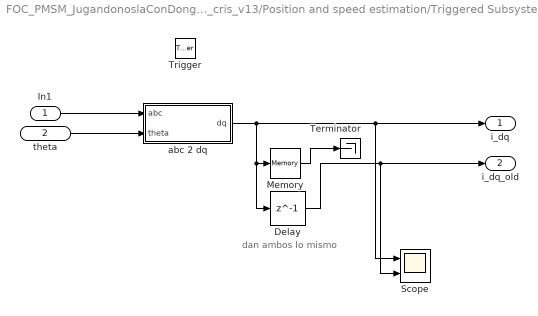
== system FOC_PMSM_JugandonoslaConDong_cris_v13/Position and speed estimation/Triggered Subsystem ==
  note: dan ambos lo mismo
  In1 : Inport
  theta : Inport  Port=2  LatchByDelayingOutsideSignal=on
  Trigger : TriggerPort  VariantControl=Variant
  Delay : Delay  DelayLength=1
  Memory : Memory  InheritSampleTime=on
  Scope : Scope  NumInputPorts=2
  Terminator : Terminator
  abc 2 dq : Subsystem
  i_dq : Outport
  i_dq_old : Outport  Port=2
  wires:
  In1/1 -> abc 2 dq/1(abc)
  abc 2 dq/1(dq) -> Delay/1, Memory/1, Scope/1, i_dq/1
  theta/1 -> abc 2 dq/2(theta)
  Delay/1 -> Scope/2, i_dq_old/1
  Memory/1 -> Terminator/1

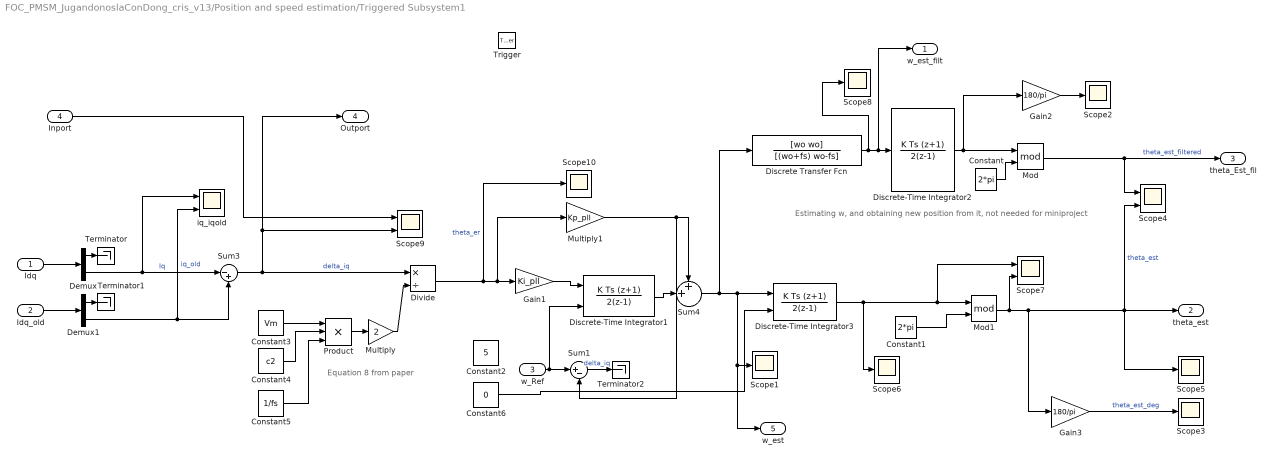
== system FOC_PMSM_JugandonoslaConDong_cris_v13/Position and speed estimation/Triggered Subsystem1 ==
  note: Estimating w, and obtaining new position from it, not needed for miniproject
  note: Equation 8 from paper
  Idq : Inport
  Idq_old : Inport  Port=2
  w_Ref : Inport  Port=3
  Inport : Inport  Port=4
  Trigger : TriggerPort  VariantControl=Variant
  Constant : Constant  Value=2*pi
  Constant1 : Constant  Value=2*pi
  Constant2 : Constant  Value=5
  Constant3 : Constant  Value=Vm
  Constant4 : Constant  Value=c2
  Constant5 : Constant  Value=1/fs
  Constant6 : Constant  Value=0
  Demux : Demux  Outputs=2
  Demux1 : Demux  Outputs=2
  Discrete Transfer Fcn : DiscreteTransferFcn  Numerator=[wo wo]  Denominator=[(wo+fs) wo-fs]
  Discrete-Time Integrator1 : DiscreteIntegrator  IntegratorMethod=Integration: Trapezoidal  gainval=1  InitialConditionSource=external  SampleTime=-1  ICPrevOutput=DiscIntNeverNeededParam  ICPrevScaledInput=DiscIntNeverNeededParam
  Discrete-Time Integrator2 : DiscreteIntegrator  IntegratorMethod=Integration: Trapezoidal  gainval=1  SampleTime=-1  ICPrevOutput=DiscIntNeverNeededParam  ICPrevScaledInput=DiscIntNeverNeededParam
  Discrete-Time Integrator3 : DiscreteIntegrator  IntegratorMethod=Integration: Trapezoidal  gainval=1  InitialConditionSource=external  SampleTime=-1  ICPrevOutput=DiscIntNeverNeededParam  ICPrevScaledInput=DiscIntNeverNeededParam
  Divide : Product  Inputs=*/
  Gain1 : Gain  Gain=Ki_pll
  Gain2 : Gain  Gain=180/pi
  Gain3 : Gain  Gain=180/pi
  Mod : Math  Operator=mod  SignedPower=off  SaturateOnIntegerOverflow=on
  Mod1 : Math  Operator=mod  SignedPower=off  SaturateOnIntegerOverflow=on
  Multiply : Gain  Gain=2
  Multiply1 : Gain  Gain=Kp_pll
  Product : Product  Inputs=3
  Scope{1..3,5..6,8,10} (7 alike) : Scope
  Scope4 : Scope  NumInputPorts=2
  Scope7 : Scope  NumInputPorts=2
  Scope9 : Scope  NumInputPorts=2
  Sum1 : Sum  Inputs=|+-
  Sum3 : Sum  Inputs=|-+
  Sum4 : Sum  Inputs=++|
  Terminator : Terminator
  Terminator1 : Terminator
  Terminator2 : Terminator
  iq_iqold : Scope  NumInputPorts=2
  w_est_filt : Outport
  theta_est : Outport  Port=2
  theta_Est_fil : Outport  Port=3
  Outport : Outport  Port=4
  w_est : Outport  Port=5
  wires:
  Discrete-Time Integrator2/1 -> Mod/1, Gain2/1
  Multiply/1 -> Divide/2
  Constant4/1 -> Product/2
  Constant5/1 -> Product/3
  Product/1 -> Multiply/1
  Gain1/1 -> Discrete-Time Integrator1/1
  Constant3/1 -> Product/1
  Gain2/1 -> Scope2/1
  Constant/1 -> Mod/2
  Discrete Transfer Fcn/1 -> Scope8/1, w_est_filt/1, Discrete-Time Integrator2/1
  Mod/1 -> theta_Est_fil/1, Scope4/1  "theta_est_filtered"
  Mod1/1 -> Scope7/2, Gain3/1, theta_est/1, Scope5/1, Scope4/2  "theta_est"
  Discrete-Time Integrator1/1 -> Sum4/2
  Constant1/1 -> Mod1/2
  Multiply1/1 -> Sum1/2, Sum4/1
  Demux/2 -> iq_iqold/1, Sum3/1  "Iq"
  Demux1/2 -> iq_iqold/2, Sum3/2  "iq_old"
  Discrete-Time Integrator3/1 -> Scope6/1, Scope7/1, Mod1/1
  Demux1/1 -> Terminator1/1
  Demux/1 -> Terminator/1
  Gain3/1 -> Scope3/1  "theta_est_deg"
  Idq_old/1 -> Demux1/1
  Idq/1 -> Demux/1
  Divide/1 -> Scope10/1, Multiply1/1, Gain1/1  "theta_er"
  Sum1/1 -> Terminator2/1  "delta_iq"
  Sum3/1 -> Scope9/2, Outport/1, Divide/1  "delta_iq"
  Inport/1 -> Scope9/1
  Constant6/1 -> Discrete-Time Integrator3/2
  w_Ref/1 -> Discrete-Time Integrator1/2, Sum1/1
  Sum4/1 -> w_est/1, Scope1/1, Discrete-Time Integrator3/1, Discrete Transfer Fcn/1

== system FOC_PMSM_JugandonoslaConDong_cris_v13/Position and speed estimation/Triggered Subsystem2 ==
  In1 : Inport
  theta : Inport  Port=2  LatchByDelayingOutsideSignal=on
  Trigger : TriggerPort  VariantControl=Variant
  Memory : Memory  InheritSampleTime=on
  abc 2 dq : Subsystem
  i_dq : Outport
  i_dq_old : Outport  Port=2
  wires:
  In1/1 -> abc 2 dq/1(abc)
  abc 2 dq/1(dq) -> Memory/1, i_dq/1
  Memory/1 -> i_dq_old/1
  theta/1 -> abc 2 dq/2(theta)

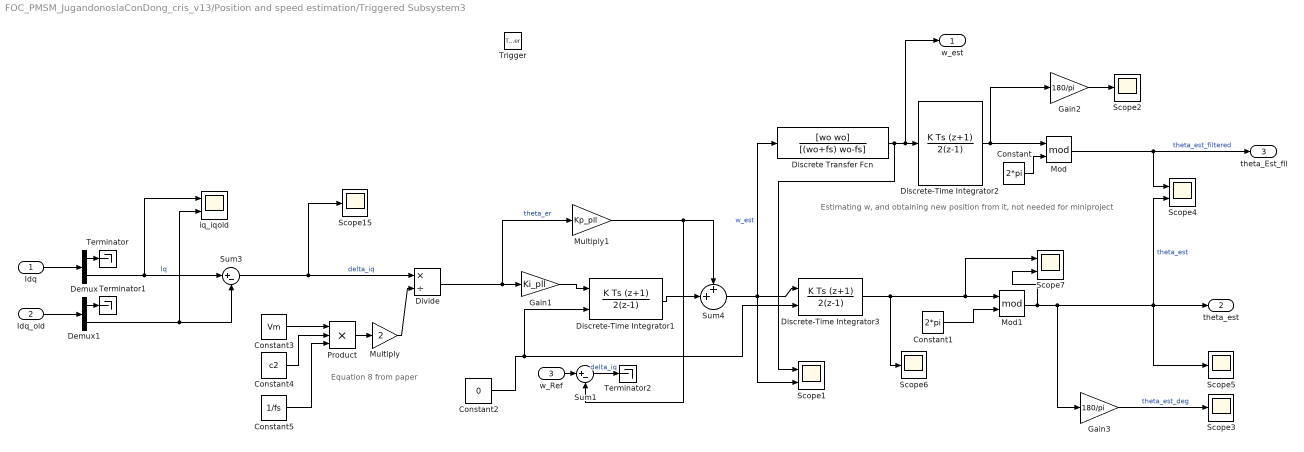
== system FOC_PMSM_JugandonoslaConDong_cris_v13/Position and speed estimation/Triggered Subsystem3 ==
  note: Estimating w, and obtaining new position from it, not needed for miniproject
  note: Equation 8 from paper
  Idq : Inport
  Idq_old : Inport  Port=2
  w_Ref : Inport  Port=3
  Trigger : TriggerPort  VariantControl=Variant
  Constant : Constant  Value=2*pi
  Constant1 : Constant  Value=2*pi
  Constant2 : Constant  Value=0
  Constant3 : Constant  Value=Vm
  Constant4 : Constant  Value=c2
  Constant5 : Constant  Value=1/fs
  Demux : Demux  Outputs=2
  Demux1 : Demux  Outputs=2
  Discrete Transfer Fcn : DiscreteTransferFcn  Numerator=[wo wo]  Denominator=[(wo+fs) wo-fs]
  Discrete-Time Integrator1 : DiscreteIntegrator  IntegratorMethod=Integration: Trapezoidal  gainval=1  InitialConditionSource=external  SampleTime=-1  ICPrevOutput=DiscIntNeverNeededParam  ICPrevScaledInput=DiscIntNeverNeededParam
  Discrete-Time Integrator2 : DiscreteIntegrator  IntegratorMethod=Integration: Trapezoidal  gainval=1  SampleTime=-1  ICPrevOutput=DiscIntNeverNeededParam  ICPrevScaledInput=DiscIntNeverNeededParam
  Discrete-Time Integrator3 : DiscreteIntegrator  IntegratorMethod=Integration: Trapezoidal  gainval=1  InitialConditionSource=external  SampleTime=-1  ICPrevOutput=DiscIntNeverNeededParam  ICPrevScaledInput=DiscIntNeverNeededParam
  Divide : Product  Inputs=*/
  Gain1 : Gain  Gain=Ki_pll
  Gain2 : Gain  Gain=180/pi
  Gain3 : Gain  Gain=180/pi
  Mod : Math  Operator=mod  SignedPower=off  SaturateOnIntegerOverflow=on
  Mod1 : Math  Operator=mod  SignedPower=off  SaturateOnIntegerOverflow=on
  Multiply : Gain  Gain=2
  Multiply1 : Gain  Gain=Kp_pll
  Product : Product  Inputs=3
  Scope1 : Scope  NumInputPorts=2
  Scope{2..3,5..6,15} (5 alike) : Scope
  Scope4 : Scope  NumInputPorts=2
  Scope7 : Scope  NumInputPorts=2
  Sum1 : Sum  Inputs=|+-
  Sum3 : Sum  Inputs=|+-
  Sum4 : Sum  Inputs=++|
  Terminator : Terminator
  Terminator1 : Terminator
  Terminator2 : Terminator
  iq_iqold : Scope  NumInputPorts=2
  w_est : Outport
  theta_est : Outport  Port=2
  theta_Est_fil : Outport  Port=3
  wires:
  Discrete-Time Integrator2/1 -> Mod/1, Gain2/1
  Multiply/1 -> Divide/2
  Constant4/1 -> Product/2
  Constant5/1 -> Product/3
  Product/1 -> Multiply/1
  Gain1/1 -> Discrete-Time Integrator1/1
  Constant3/1 -> Product/1
  Gain2/1 -> Scope2/1
  Constant/1 -> Mod/2
  Discrete Transfer Fcn/1 -> Scope1/1, w_est/1, Discrete-Time Integrator2/1
  Mod/1 -> theta_Est_fil/1, Scope4/1  "theta_est_filtered"
  Mod1/1 -> Scope7/2, Gain3/1, theta_est/1, Scope5/1, Scope4/2  "theta_est"
  Discrete-Time Integrator1/1 -> Sum4/2
  Constant1/1 -> Mod1/2
  Sum4/1 -> Scope1/2, Discrete Transfer Fcn/1, Discrete-Time Integrator3/1  "w_est"
  Multiply1/1 -> Sum1/2, Sum4/1
  Sum3/1 -> Scope15/1, Divide/1  "delta_iq"
  Demux/2 -> iq_iqold/1, Sum3/1  "Iq"
  Demux1/2 -> iq_iqold/2, Sum3/2
  Discrete-Time Integrator3/1 -> Scope6/1, Scope7/1, Mod1/1
  Demux1/1 -> Terminator1/1
  Demux/1 -> Terminator/1
  Gain3/1 -> Scope3/1  "theta_est_deg"
  Idq_old/1 -> Demux1/1
  Idq/1 -> Demux/1
  w_Ref/1 -> Sum1/1
  Divide/1 -> Multiply1/1, Gain1/1  "theta_er"
  Constant2/1 -> Discrete-Time Integrator1/2, Discrete-Time Integrator3/2
  Sum1/1 -> Terminator2/1  "delta_iq"

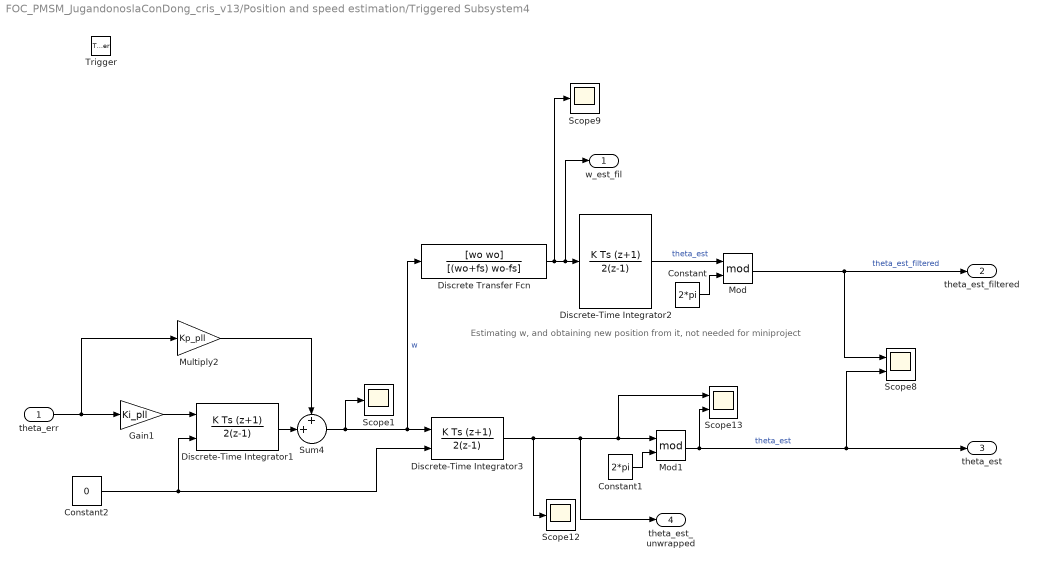
== system FOC_PMSM_JugandonoslaConDong_cris_v13/Position and speed estimation/Triggered Subsystem4 ==
  note: Estimating w, and obtaining new position from it, not needed for miniproject
  theta_err : Inport
  Trigger : TriggerPort  VariantControl=Variant
  Constant : Constant  Value=2*pi
  Constant1 : Constant  Value=2*pi
  Constant2 : Constant  Value=0
  Discrete Transfer Fcn : DiscreteTransferFcn  Numerator=[wo wo]  Denominator=[(wo+fs) wo-fs]
  Discrete-Time Integrator1 : DiscreteIntegrator  IntegratorMethod=Integration: Trapezoidal  gainval=1  InitialConditionSource=external  SampleTime=-1  ICPrevOutput=DiscIntNeverNeededParam  ICPrevScaledInput=DiscIntNeverNeededParam
  Discrete-Time Integrator2 : DiscreteIntegrator  IntegratorMethod=Integration: Trapezoidal  gainval=1  SampleTime=-1  ICPrevOutput=DiscIntNeverNeededParam  ICPrevScaledInput=DiscIntNeverNeededParam
  Discrete-Time Integrator3 : DiscreteIntegrator  IntegratorMethod=Integration: Trapezoidal  gainval=1  InitialConditionSource=external  SampleTime=-1  ICPrevOutput=DiscIntNeverNeededParam  ICPrevScaledInput=DiscIntNeverNeededParam
  Gain1 : Gain  Gain=Ki_pll
  Mod : Math  Operator=mod  SignedPower=off  SaturateOnIntegerOverflow=on
  Mod1 : Math  Operator=mod  SignedPower=off  SaturateOnIntegerOverflow=on
  Multiply2 : Gain  Gain=Kp_pll
  Scope1 : Scope
  Scope12 : Scope
  Scope13 : Scope  NumInputPorts=2
  Scope8 : Scope  NumInputPorts=2
  Scope9 : Scope
  Sum4 : Sum  Inputs=++|
  w_est_fil : Outport
  theta_est_filtered : Outport  Port=2
  theta_est : Outport  Port=3
  theta_est_unwrapped : Outport  Port=4
  wires:
  Gain1/1 -> Discrete-Time Integrator1/1
  Multiply2/1 -> Sum4/1
  Mod/1 -> theta_est_filtered/1, Scope8/1  "theta_est_filtered"
  Sum4/1 -> Discrete Transfer Fcn/1, Discrete-Time Integrator3/1, Scope1/1  "w"
  Mod1/1 -> Scope13/2, Scope8/2, theta_est/1  "theta_est"
  Constant2/1 -> Discrete-Time Integrator3/2, Discrete-Time Integrator1/2
  Constant/1 -> Mod/2
  Discrete-Time Integrator3/1 -> Scope12/1, theta_est_unwrapped/1, Scope13/1, Mod1/1
  Discrete-Time Integrator1/1 -> Sum4/2
  Discrete Transfer Fcn/1 -> Scope9/1, w_est_fil/1, Discrete-Time Integrator2/1
  Constant1/1 -> Mod1/2
  Discrete-Time Integrator2/1 -> Mod/1  "theta_est"
  theta_err/1 -> Multiply2/1, Gain1/1

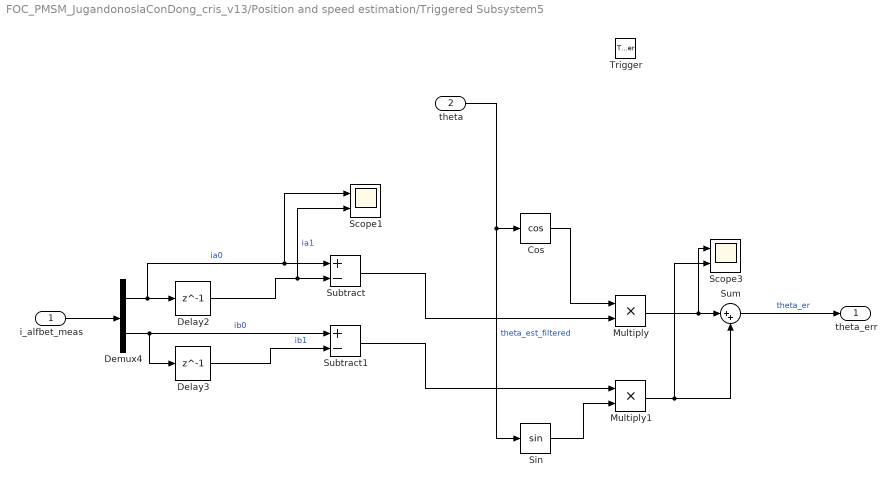
== system FOC_PMSM_JugandonoslaConDong_cris_v13/Position and speed estimation/Triggered Subsystem5 ==
  i_alfbet_meas : Inport
  theta : Inport  Port=2  LatchByDelayingOutsideSignal=on
  Trigger : TriggerPort  VariantControl=Variant
  Cos : Trigonometry  Operator=cos
  Delay2 : Delay  DelayLength=1
  Delay3 : Delay  DelayLength=1
  Demux4 : Demux  Outputs=2
  Multiply : Product
  Multiply1 : Product
  Scope1 : Scope  NumInputPorts=2
  Scope3 : Scope  NumInputPorts=2
  Sin : Trigonometry
  Subtract : Sum  Inputs=+-
  Subtract1 : Sum  Inputs=+-
  Sum : Sum  Inputs=|++
  theta_err : Outport
  wires:
  Cos/1 -> Multiply/1
  Sum/1 -> theta_err/1  "theta_er"
  Sin/1 -> Multiply1/2
  Demux4/1 -> Scope1/1, Subtract/1, Delay2/1  "ia0"
  Multiply1/1 -> Sum/2, Scope3/2
  Delay3/1 -> Subtract1/2  "ib1"
  Demux4/2 -> Delay3/1, Subtract1/1  "ib0"
  i_alfbet_meas/1 -> Demux4/1
  Subtract/1 -> Multiply/2
  theta/1 -> Sin/1, Cos/1  "theta_est_filtered"
  Subtract1/1 -> Multiply1/1
  Multiply/1 -> Scope3/1, Sum/1
  Delay2/1 -> Scope1/2, Subtract/2  "ia1"

== system FOC_PMSM_JugandonoslaConDong_cris_v13/Position and speed estimation/Triggered Subsystem/abc 2 dq ==
  abc : Inport
  theta : Inport  Port=2
  Mux1 : Mux  Inputs=2
  Mux2 : Mux  Inputs=2
  abc2d : Fcn  Expr=2/3*(u(1)*cos(u(4))+u(2)*cos(u(4)-2*pi/3)+u(3)*cos(u(4)-4*pi/3))
  abc2q : Fcn  Expr=-1*2/3*(u(1)*sin(u(4))+u(2)*sin(u(4)-2*pi/3)+u(3)*sin(u(4)-4*pi/3))
  dq : Outport  VectorParamsAs1DForOutWhenUnconnected=off
  wires:
  Mux2/1 -> dq/1
  abc2q/1 -> Mux2/2
  abc2d/1 -> Mux2/1
  Mux1/1 -> abc2q/1, abc2d/1
  theta/1 -> Mux1/2
  abc/1 -> Mux1/1

== system FOC_PMSM_JugandonoslaConDong_cris_v13/Position and speed estimation/Triggered Subsystem2/abc 2 dq ==
  abc : Inport
  theta : Inport  Port=2
  Mux1 : Mux  Inputs=2
  Mux2 : Mux  Inputs=2
  abc2d : Fcn  Expr=2/3*(u(1)*cos(u(4))+u(2)*cos(u(4)-2*pi/3)+u(3)*cos(u(4)-4*pi/3))
  abc2q : Fcn  Expr=-1*2/3*(u(1)*sin(u(4))+u(2)*sin(u(4)-2*pi/3)+u(3)*sin(u(4)-4*pi/3))
  dq : Outport  VectorParamsAs1DForOutWhenUnconnected=off
  wires:
  Mux2/1 -> dq/1
  abc2q/1 -> Mux2/2
  abc2d/1 -> Mux2/1
  Mux1/1 -> abc2q/1, abc2d/1
  theta/1 -> Mux1/2
  abc/1 -> Mux1/1
